simulink model "MNIST_simulink"  (R2024a)
settings: Solver=VariableStepAuto  StartTime=0.0  StopTime=10.0  RelTol=1e-3
undefined symbols (not defined in the file or in its folder): Rec, SDTV
libraries: visionconversions x1, visionsources x1, deeplib x1
settings Model: Creator=rerse  LastModifiedBy=rerse

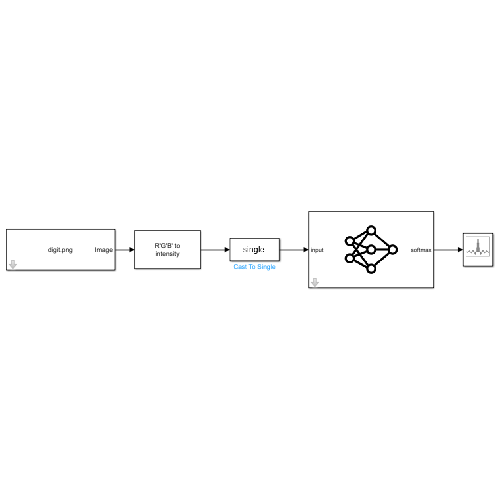
[thumbnail: Simulink's stored preview of the top-level diagram]
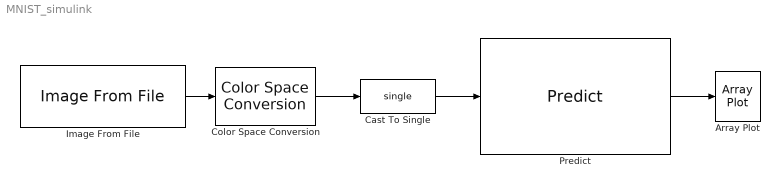
== system MNIST_simulink ==
  Array Plot : ArrayPlot  WindowPosition=[560.000000,290.000000,800.000000,500.000000,]  ScopeFrameLocation=window  YLimits=[-0.1237 1.1133]
  Cast To Single : DataTypeConversion  OutDataTypeStr=single  SaturateOnIntegerOverflow=off  RndMeth=Floor
  Color Space Conversion : visionconversions/Color Space  Conversion  conversion=Obsolete  conversionActive=R'G'B' to intensity  wp_str=D65  rec=Rec. 601 (SDTV)  sys=1125/60/2:1  imagePorts=One multidimensional signal
  Image From File : visionsources/Image From File  Tag=vipblks_nd  FileName=C:\Users\rerse\MATLAB\Projects\MNIST\digit.png  Ts=inf  imagePorts=One multidimensional signal  OutPortLabels=R|G|B  ImageDataType=Inherit from input image  sdImageDataType=uint(8)  Signed=on  WordLength=16  FractionLengthMode=User-defined  FractionLength=15
  Predict : deeplib/Predict  Network=Network from MAT-file  NetworkFunction=squeezenet  NetworkFilePath=C:\Users\rerse\MATLAB\Projects\MNIST\trained_mnist_model.mat  MiniBatchSize=128  InputDataFormats={ 'input', 'SSCB' }  Predictions=on  Activations={}  ForceInterpretedSim=off  EnableDLNetwork=on  LastKnownNetworkFilePath='C:\Users\rerse\MATLAB\Projects\MNIST\trained_mnist_model.mat'  LastKnownNetworkTimeStamp=740064.49996527773328125476837158203125
  wires:
  Image From File/1 -> Color Space Conversion/1
  Color Space Conversion/1 -> Cast To Single/1
  Cast To Single/1 -> Predict/1
  Predict/1 -> Array Plot/1
